simulink model "basic_FC"  (R2023b)
settings: Solver=VariableStepAuto  StartTime=0.0  StopTime=3600*8760*3  MaxStep=1000  RelTol=1e-5
values from neighbouring files (symbols this model uses):
  I_s_0 = 1.85    [fuelCycleSimulator.m]    (also in parametric_analysis_AF.m = 0.8; parametric_analysis_epsi.m = 0.8; parametric_analysis_eta_tes.m = 0.8; parametric_analysis_f_dir.m = 0.8)
  N_dot = 8.99e-7    (= 8.99e-07)    [BOTH_scenario_inputData.m]    (also in FC_scenario_inputData.m = 9.3e-07; PO_scenario_inputData.m = 9.3e-07; inputData.m = 9.3e-07; worst_case_InputData.m = 9.3e-07)
  TBE = 0.1    [BOTH_scenario_inputData.m]    (also in FC_scenario_inputData.m = 0.02; PO_scenario_inputData.m; inputData.m = 0.02; parametric_analysis_AF.m = TBE_array(j))
  TBR = 1.096    [fuelCycleSimulator.m]    (also in parametric_analysis_AF.m = 1; parametric_analysis_TBE.m = 1; parametric_analysis_epsi.m = 1; parametric_analysis_eta_tes.m = 1)
undefined symbols (not defined in the file or in its folder): arc, fuelCleanUp_8, storage_10, tau_ifc, tau_ofc
settings Model: Creator=smesc  LastModifiedBy=meschini
settings SolverCC: InitialStep=1e-4
settings ModelReferenceCC: EnableRefExpFcnMdlSchedulingChecks=on

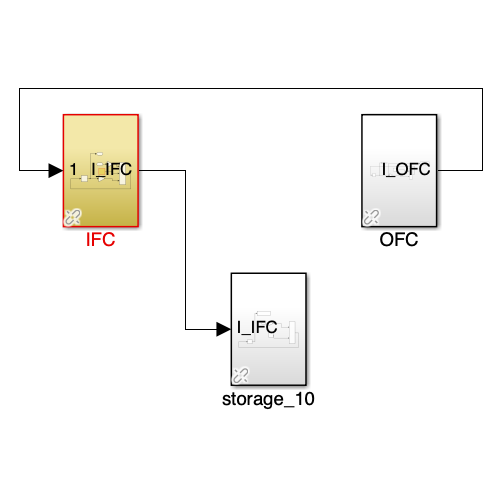
[thumbnail: Simulink's stored preview of the top-level diagram]
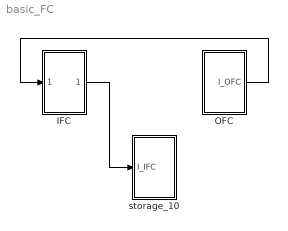
== system basic_FC ==
  IFC : Subsystem  AncestorBlock=arc/fuelCleanUp_8
  OFC : Subsystem  AncestorBlock=arc/fuelCleanUp_8
  storage_10 : Subsystem  AncestorBlock=arc/storage_10
  wires:
  OFC/1(I_OFC) -> IFC/1(Input)
  IFC/1(I_IFC) -> storage_10/1(I_IFC)

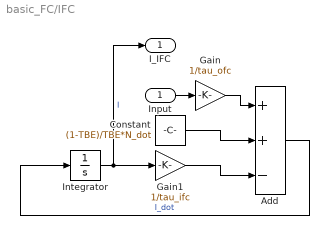
== system basic_FC/IFC ==
  Input : Inport
  Add : Sum  Inputs=++-
  Constant : Constant  Value=(1-TBE)/TBE*N_dot
  Gain : Gain  Gain=1/tau_ofc
  Gain1 : Gain  Gain=1/tau_ifc
  Integrator : Integrator
  I_IFC : Outport
  wires:
  Input/1 -> Gain/1
  Add/1 -> Integrator/1  "I_dot"
  Integrator/1 -> Gain1/1, I_IFC/1  "I"
  Gain/1 -> Add/1
  Gain1/1 -> Add/3
  Constant/1 -> Add/2

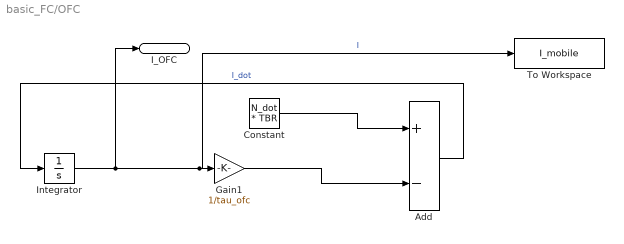
== system basic_FC/OFC ==
  Add : Sum  Inputs=+-
  Constant : Constant  Value=N_dot * TBR
  Gain1 : Gain  Gain=1/tau_ofc
  Integrator : Integrator
  To Workspace : ToWorkspace  VariableName=I_mobile  SampleTime=-1
  I_OFC : Outport
  wires:
  Gain1/1 -> Add/2
  Add/1 -> Integrator/1  "I_dot"
  Integrator/1 -> To Workspace/1, Gain1/1, I_OFC/1  "I"
  Constant/1 -> Add/1

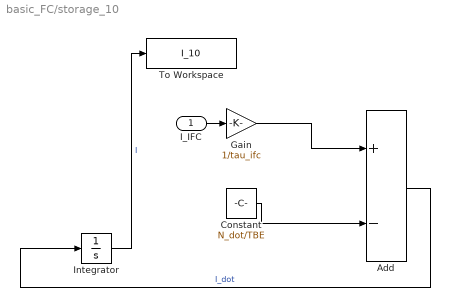
== system basic_FC/storage_10 ==
  I_IFC : Inport
  Add : Sum  Inputs=+-
  Constant : Constant  Value=N_dot/TBE
  Gain : Gain  Gain=1/tau_ifc
  Integrator : Integrator  InitialCondition=I_s_0
  To Workspace : ToWorkspace  VariableName=I_10  SampleTime=-1
  wires:
  Integrator/1 -> To Workspace/1  "I"
  Add/1 -> Integrator/1  "I_dot"
  Constant/1 -> Add/2
  I_IFC/1 -> Gain/1
  Gain/1 -> Add/1
